simulink model "scon2_L9_1ponto1_simulink"  (R2024a)
settings: Solver=VariableStepAuto  StartTime=0.0  StopTime=10.0  RelTol=1e-3
values from neighbouring files (symbols this model uses):
  A = [1, 2; -6, -12]    [scon2_L9_1ponto1.m]
  B = [-5; 1]    [scon2_L9_1ponto1.m]
  C = [4, -3]    [scon2_L9_1ponto1.m]
  K = acker(A, B, J_c)    [scon2_L9_1ponto1.m]
  K_e = acker(A', C', J_o)'    [scon2_L9_1ponto1.m]
  x0 = [1; 2]    [scon2_L9_1ponto1.m]
  x0_o = [1; 0]    [scon2_L9_1ponto1.m]
settings Model: Creator=Carlos Augusto  LastModifiedBy=Carlos Augusto

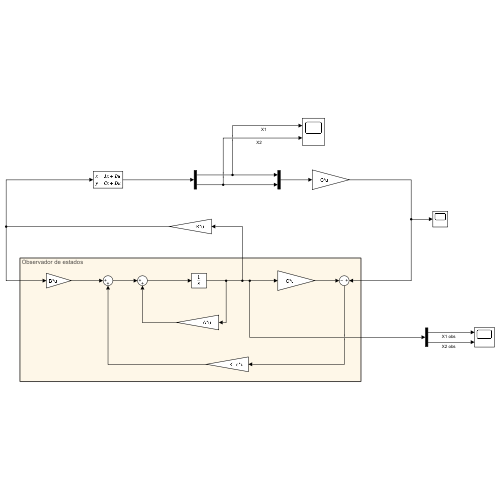
[thumbnail: Simulink's stored preview of the top-level diagram]
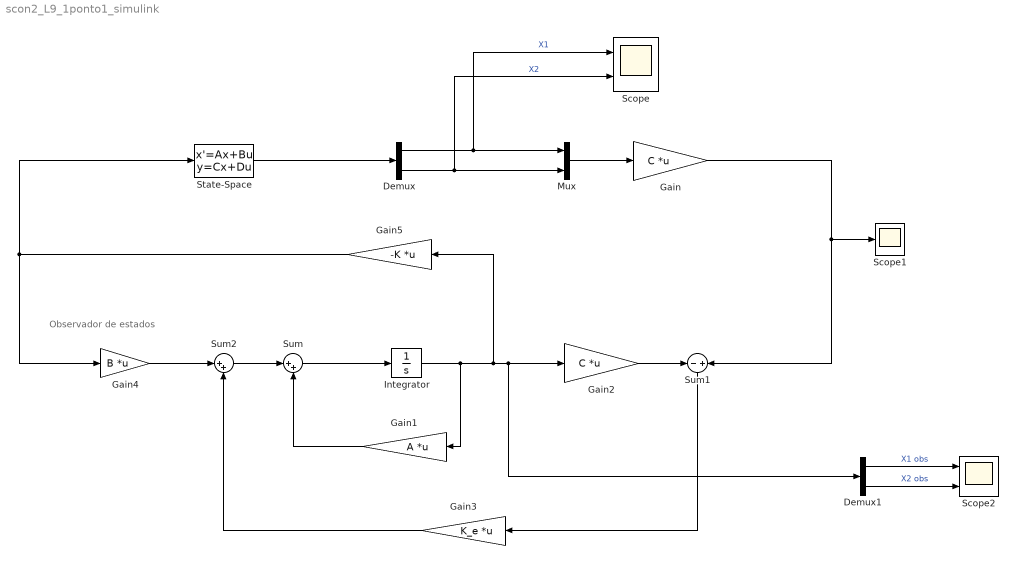
== system scon2_L9_1ponto1_simulink ==
  note: Observador de estados
  Demux : Demux  Outputs=2
  Demux1 : Demux  Outputs=2
  Gain : Gain  Gain=C  Multiplication=Matrix(K*u)
  Gain1 : Gain  Gain=A  Multiplication=Matrix(K*u)
  Gain2 : Gain  Gain=C  Multiplication=Matrix(K*u)
  Gain3 : Gain  Gain=K_e  Multiplication=Matrix(K*u)
  Gain4 : Gain  Gain=B  Multiplication=Matrix(K*u)
  Gain5 : Gain  Gain=-K  Multiplication=Matrix(K*u)
  Integrator : Integrator  InitialCondition=x0_o
  Mux : Mux  Inputs=2
  Scope : Scope  NumInputPorts=2
  Scope1 : Scope
  Scope2 : Scope  NumInputPorts=2
  State-Space : StateSpace  A=A  B=B  C=eye(2)  D=zeros(2,1)  InitialCondition=x0
  Sum : Sum  Inputs=|++
  Sum1 : Sum  Inputs=-+
  Sum2 : Sum  Inputs=|++
  wires:
  Integrator/1 -> Gain5/1, Demux1/1, Gain2/1, Gain1/1
  Sum/1 -> Integrator/1
  Demux1/2 -> Scope2/2  "X2 obs"
  State-Space/1 -> Demux/1
  Demux/2 -> Mux/2, Scope/2  "X2"
  Sum2/1 -> Sum/1
  Gain/1 -> Scope1/1, Sum1/2
  Demux1/1 -> Scope2/1  "X1 obs"
  Gain5/1 -> Gain4/1, State-Space/1
  Gain4/1 -> Sum2/1
  Gain3/1 -> Sum2/2
  Gain1/1 -> Sum/2
  Sum1/1 -> Gain3/1
  Demux/1 -> Mux/1, Scope/1  "X1"
  Mux/1 -> Gain/1
  Gain2/1 -> Sum1/1
